simulink model "DUST4_Nonlinear_Airframe"  (R2024b)
settings: Solver=VariableStepAuto  StartTime=0.0  StopTime=10.0  RelTol=1e-3
undefined symbols (not defined in the file or in its folder): AC, Aero, mot, prop, rad, s, Vbi
libraries: aerolibasang x3, aerolibconvert2 x3, aerolibactuator x3, shared6dof x2, aerolibtransform2 x2, aerolibadyn x1, vrlib x1
(part 1 of 2)
settings Model: DataDictionary=DUST4_Airframe.sldd  Creator=Tristan  LastModifiedBy=theon

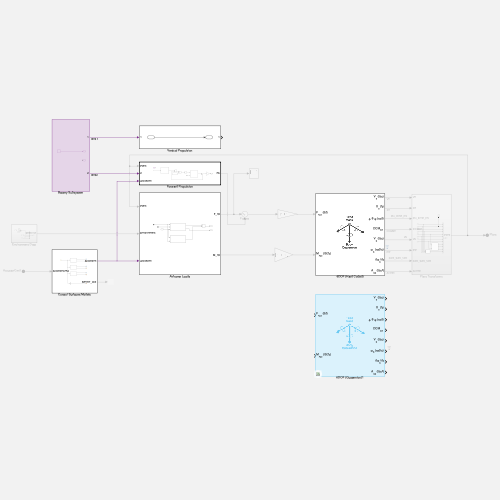
[thumbnail: Simulink's stored preview of the top-level diagram]
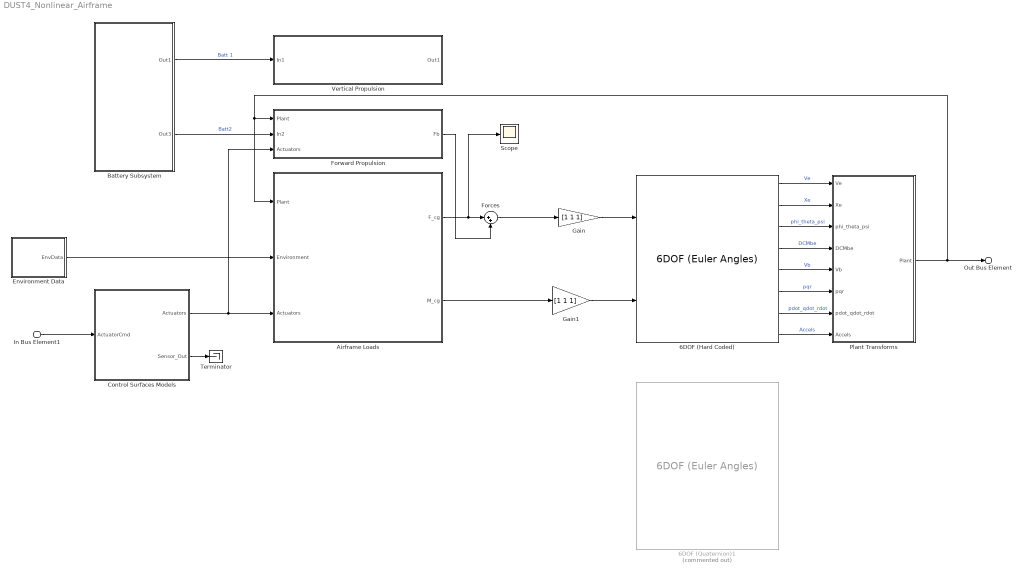
== system DUST4_Nonlinear_Airframe ==
  In Bus Element1 : Inport  PortName=ActuatorCmd
  6DOF (Hard Coded) : shared6dof/6DOF (Euler Angles)  units=English (Velocity in ft/s)  mtype=Fixed  rep=Quaternion  xme_0=[0 0 0]  Vm_0=[0 0 0]  eul_0=[0 0 0]  pm_0=[0 0 0]  mass_0=0.115  mass_e=0.5  mass_f=2.0  inertia=diag([11.38 9.6 20.40])  inertia_e=eye(3)  inertia_f=2*eye(3)  k_quat=1.0  vre_flag=on  abi_flag=off  aMode=0  xme_statename=''  Vm_statename=''  eul_statename=''  quat_statename=''  pm_statename=''  mass_statename=''
  6DOF (Quaternion)1 : shared6dof/6DOF (Euler Angles)  Commented=on  units=English (Velocity in ft/s)  mtype=Fixed  rep=Quaternion  xme_0=[0 0 0]  Vm_0=Vbi  eul_0=[0 0 0]  pm_0=[0 0 0]  mass_0=AC.mass  mass_e=0.5  mass_f=2.0  inertia=AC.Inertia  inertia_e=eye(3)  inertia_f=2*eye(3)  k_quat=1.0  vre_flag=on  abi_flag=off  aMode=0  xme_statename=''  Vm_statename=''  eul_statename=''  quat_statename=''  pm_statename=''  mass_statename=''
  Airframe Loads : Subsystem
  Battery Subsystem : Subsystem
  Control Surfaces Models : Subsystem
  Environment Data : Subsystem
  Forces : Sum  Inputs=|++
  Forward Propulsion : Subsystem  TreatAsAtomicUnit=on
  Gain : Gain  Gain=[1 1 1]
  Gain1 : Gain  Gain=[1 1 1]
  Plant Transforms : Subsystem
  Scope : Scope
  Terminator : Terminator
  Vertical Propulsion : Subsystem
  Out Bus Element : Outport  PortName=Plant
  wires:
  Forces/1 -> Gain/1
  6DOF (Hard Coded)/7 -> Plant Transforms/7(pdot_qdot_rdot)  "pdot_qdot_rdot"
  6DOF (Hard Coded)/2 -> Plant Transforms/2(Xe)  "Xe"
  6DOF (Hard Coded)/6 -> Plant Transforms/6(pqr)  "pqr"
  Airframe Loads/1(F_cg) -> Scope/1, Forces/1
  6DOF (Hard Coded)/5 -> Plant Transforms/5(Vb)  "Vb"
  In Bus Element1/1 -> Control Surfaces Models/1(ActuatorCmd)
  Environment Data/1(EnvData) -> Airframe Loads/2(Environment)
  Plant Transforms/1(Plant) -> Out Bus Element/1, Airframe Loads/1(Plant), Forward Propulsion/1(Plant)
  6DOF (Hard Coded)/3 -> Plant Transforms/3(phi_theta_psi)  "phi_theta_psi"
  6DOF (Hard Coded)/8 -> Plant Transforms/8(Accels)  "Accels"
  6DOF (Hard Coded)/1 -> Plant Transforms/1(Ve)  "Ve"
  Airframe Loads/2(M_cg) -> Gain1/1
  Gain/1 -> 6DOF (Hard Coded)/1
  Forward Propulsion/1(Fb) -> Forces/2
  6DOF (Hard Coded)/4 -> Plant Transforms/4(DCMbe)  "DCMbe"
  Control Surfaces Models/2(Sensor_Out) -> Terminator/1
  Gain1/1 -> 6DOF (Hard Coded)/2
  Battery Subsystem/2(Out3) -> Forward Propulsion/2(In2)  "Batt2"
  Battery Subsystem/1(Out1) -> Vertical Propulsion/1(In1)  "Batt 1"
  Control Surfaces Models/1(Actuators) -> Airframe Loads/3(Actuators), Forward Propulsion/3(Actuators)

== system DUST4_Nonlinear_Airframe/Airframe Loads ==
  Plant : Inport
  In Bus Element : Inport  Port=2  PortName=Environment
  In Bus Element1 : Inport  Port=3  PortName=Actuators
  Add : Sum
  Aerodynamic Loads : Subsystem
  Gravity Force : Subsystem
  F_cg : Outport
  M_cg : Outport  Port=2
  wires:
  Plant/1 -> Gravity Force/1(Plant), Aerodynamic Loads/3(plant)
  In Bus Element/1 -> Gravity Force/2(Environment), Aerodynamic Loads/1(EnvData)
  In Bus Element1/1 -> Aerodynamic Loads/2(Actuators)
  Aerodynamic Loads/1(Fb) -> Add/1
  Add/1 -> F_cg/1
  Aerodynamic Loads/2(Mb) -> M_cg/1
  Gravity Force/1(Fg_b) -> Add/2

== system DUST4_Nonlinear_Airframe/Battery Subsystem ==
  Initial Voltage : Constant
  Out1 : Outport
  Out3 : Outport  Port=2
  wires:
  Initial Voltage/1 -> Out1/1

== system DUST4_Nonlinear_Airframe/Control Surfaces Models ==
  In Bus Element1 : Inport  PortName=ActuatorCmd
  Ailerons : Subsystem
  Bus Selector : BusSelector  OutputSignals=Throttle
  Elevator : Subsystem
  Rudder : Subsystem
  Out Bus Element2 : Outport  VectorParamsAs1DForOutWhenUnconnected=off  PortName=Actuators  Element=Aileron
  Out Bus Element3 : Outport  VectorParamsAs1DForOutWhenUnconnected=off  PortName=Actuators  Element=Elevator
  Out Bus Element4 : Outport  VectorParamsAs1DForOutWhenUnconnected=off  PortName=Actuators  Element=Rudder
  BusElementOut : Outport  PortName=Actuators  Element=Throttle
  Out Bus Element12 : Outport  Port=2  VectorParamsAs1DForOutWhenUnconnected=off  PortName=Sensor_Out  Element=Ail
  Out Bus Element1 : Outport  Port=2  VectorParamsAs1DForOutWhenUnconnected=off  PortName=Sensor_Out  Element=Ele
  Out Bus Element5 : Outport  Port=2  VectorParamsAs1DForOutWhenUnconnected=off  PortName=Sensor_Out  Element=Rud
  wires:
  Ailerons/1(SensorOut) -> Out Bus Element12/1  "Rudder"
  Ailerons/2(Positions) -> Out Bus Element2/1  "Rudder"
  In Bus Element1/1 -> Bus Selector/1, Rudder/1(Commands), Elevator/1(Commands), Ailerons/1(Commands)
  Elevator/1(SensorOut) -> Out Bus Element1/1  "Rudder"
  Elevator/2(Positions) -> Out Bus Element3/1  "Rudder"
  Rudder/2(Positions) -> Out Bus Element4/1  "Rudder"
  Rudder/1(SensorOut) -> Out Bus Element5/1  "Rudder"
  Bus Selector/1 -> BusElementOut/1  "<Throttle>"

== system DUST4_Nonlinear_Airframe/Environment Data ==
  Air Density : Constant  Value=0.002377
  Bus Creator : BusCreator  Inputs=5
  Constant : Constant  Value=0
  Constant1 : Constant  Value=0
  Constant2 : Constant  Value=32.2
  Gravity Acceleration : Constant  Value=[0 0 32.2]
  Mux : Mux  Inputs=3
  Speed of Sound : Constant  Value=1100
  Wind Angular Rates : Constant  Value=[0 0 0]
  Wind Velocity : Constant  Value=[0 0 0]
  EnvData : Outport
  wires:
  Air Density/1 -> Bus Creator/3  "rho"
  Speed of Sound/1 -> Bus Creator/2  "a"
  Mux/1 -> Bus Creator/1  "Ag"
  Wind Velocity/1 -> Bus Creator/4  "WindVelocity"
  Wind Angular Rates/1 -> Bus Creator/5  "WindAngularRates"
  Bus Creator/1 -> EnvData/1  "Environment"
  Constant/1 -> Mux/1
  Constant1/1 -> Mux/2
  Constant2/1 -> Mux/3

== system DUST4_Nonlinear_Airframe/Forward Propulsion ==
  In Bus Element2 : Inport  PortName=Plant  Element=Airspeed
  In2 : Inport  Port=2
  In Bus Element1 : Inport  Port=3  PortName=Actuators  Element=Throttle
  Bus Selector1 : BusSelector  OutputSignals=Thrust,Torque
  Divide1 : Product  Inputs=*/
  Gain1 : Gain  Gain=[1 0 0]
  Integrator : Integrator  InitialCondition=200
  Motor Model : Subsystem
  Prop MOI (slug-ft^2) : Constant  Value=prop.MOI
  Propeller Model : Subsystem
  Subtract : Sum  Inputs=+-
  Fb : Outport
  wires:
  In Bus Element2/1 -> Propeller Model/2(Airspeed)
  Propeller Model/1(Propulsion Data) -> Bus Selector1/1
  Prop MOI (slug-ft^2)/1 -> Divide1/2
  Divide1/1 -> Integrator/1  "Omega dot"
  In Bus Element1/1 -> Motor Model/1(Throttle)
  Integrator/1 -> Propeller Model/1(Omega)  "omega"
  Subtract/1 -> Divide1/1
  Motor Model/1(Torque (ft-lbf)) -> Subtract/1
  Bus Selector1/2 -> Subtract/2  "<Torque>"
  Bus Selector1/1 -> Gain1/1  "<Thrust>"
  Gain1/1 -> Fb/1

== system DUST4_Nonlinear_Airframe/Plant Transforms ==
  Ve : Inport
  Xe : Inport  Port=2
  phi_theta_psi : Inport  Port=3
  DCMbe : Inport  Port=4
  Vb : Inport  Port=5
  pqr : Inport  Port=6
  pdot_qdot_rdot : Inport  Port=7
  Accels : Inport  Port=8
  ModelBus : BusCreator  Inputs=12
  Scope : Scope
  Subsystem1 : Subsystem
  WingConnectorPlant : Subsystem
  Plant : Outport
  wires:
  Ve/1 -> WingConnectorPlant/2(Ve), ModelBus/1  "Ve"
  ModelBus/1 -> Plant/1
  DCMbe/1 -> ModelBus/4, WingConnectorPlant/1(DCMbe)  "DCMbe"
  pqr/1 -> WingConnectorPlant/4(pqr), ModelBus/6  "pqr"
  pdot_qdot_rdot/1 -> ModelBus/7  "pdot_qdot_rdot"
  Subsystem1/2("alpha_dot, beta_dot") -> ModelBus/10  "alphadot_betadot"
  WingConnectorPlant/1(WingConnector) -> ModelBus/12  "AC1_Connector"
  Xe/1 -> WingConnectorPlant/3(Xe), ModelBus/2, Scope/1  "Xe"
  Subsystem1/1("alpha, beta") -> ModelBus/9  "alpha_beta"
  phi_theta_psi/1 -> ModelBus/3  "phi_theta_psi"
  Accels/1 -> Subsystem1/2(Ab), ModelBus/8  "Ab"
  Vb/1 -> Subsystem1/1(Vb), ModelBus/5  "Vb"
  Subsystem1/3(Airspeed) -> ModelBus/11  "Airspeed"

== system DUST4_Nonlinear_Airframe/Vertical Propulsion ==
  In1 : Inport
  Out1 : Outport
  wires:
  In1/1 -> Out1/1

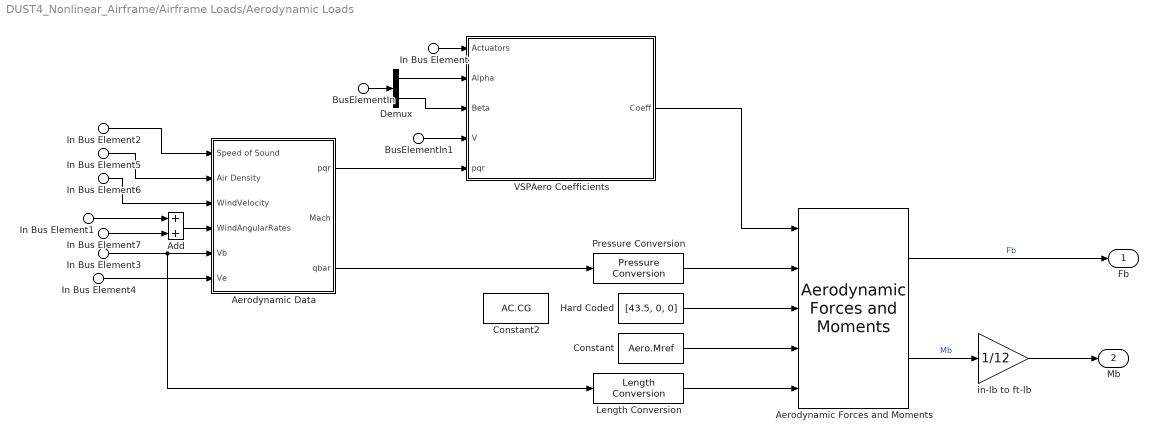
== system DUST4_Nonlinear_Airframe/Airframe Loads/Aerodynamic Loads ==
  In Bus Element6 : Inport  PortName=EnvData  Element=WindVelocity
  In Bus Element7 : Inport  PortName=EnvData  Element=WindAngularRates
  In Bus Element2 : Inport  PortName=EnvData  Element=a
  In Bus Element5 : Inport  PortName=EnvData  Element=rho
  In Bus Element : Inport  Port=2  PortName=Actuators
  In Bus Element3 : Inport  Port=3  PortName=plant  Element=Vb
  In Bus Element4 : Inport  Port=3  PortName=plant  Element=Ve
  In Bus Element1 : Inport  Port=3  PortName=plant  Element=pqr
  BusElementIn : Inport  Port=3  PortName=plant  Element=alpha_beta
  BusElementIn1 : Inport  Port=3  PortName=plant  Element=Airspeed
  Add : Sum
  Aerodynamic Forces and Moments : aerolibadyn/Aerodynamic Forces and Moments   inputAxes=Wind  outputForceAxes=Body  outputMomentAxes=Body  S=Aero.Sref  b=Aero.bref  cbar=Aero.Cref
  Aerodynamic Data : Subsystem
  Constant : Constant  Value=Aero.Mref
  Constant2 : Constant  Value=AC.CG
  Demux : Demux  Outputs=2
  Hard Coded : Constant  Value=[43.5, 0, 0]
  Length Conversion : aerolibconvert2/Length Conversion  IU=ft  OU=in
  Pressure Conversion : aerolibconvert2/Pressure Conversion  IU=psf  OU=psi
  VSPAero Coefficients : Subsystem
  in-lb to ft-lb : Gain  Gain=1/12
  Fb : Outport  VectorParamsAs1DForOutWhenUnconnected=off
  Mb : Outport  Port=2  VectorParamsAs1DForOutWhenUnconnected=off
  wires:
  In Bus Element6/1 -> Aerodynamic Data/3(WindVelocity)
  Aerodynamic Data/1("pqr ") -> VSPAero Coefficients/5(pqr)
  Aerodynamic Forces and Moments/2 -> in-lb to ft-lb/1  "Mb"
  VSPAero Coefficients/1(Coeff) -> Aerodynamic Forces and Moments/1
  In Bus Element7/1 -> Add/2
  Constant/1 -> Aerodynamic Forces and Moments/4
  In Bus Element5/1 -> Aerodynamic Data/2(Air Density)
  In Bus Element2/1 -> Aerodynamic Data/1(Speed of Sound)
  Add/1 -> Aerodynamic Data/4(WindAngularRates)
  In Bus Element4/1 -> Aerodynamic Data/6(Ve)
  Aerodynamic Forces and Moments/1 -> Fb/1  "Fb"
  In Bus Element1/1 -> Add/1
  In Bus Element/1 -> VSPAero Coefficients/1(Actuators)
  BusElementIn1/1 -> VSPAero Coefficients/4(V)
  BusElementIn/1 -> Demux/1
  Demux/1 -> VSPAero Coefficients/2(Alpha)
  Demux/2 -> VSPAero Coefficients/3(Beta)
  In Bus Element3/1 -> Length Conversion/1, Aerodynamic Data/5(Vb)
  Aerodynamic Data/3(qbar) -> Pressure Conversion/1
  Hard Coded/1 -> Aerodynamic Forces and Moments/3
  Pressure Conversion/1 -> Aerodynamic Forces and Moments/2
  Length Conversion/1 -> Aerodynamic Forces and Moments/5
  in-lb to ft-lb/1 -> Mb/1

== system DUST4_Nonlinear_Airframe/Airframe Loads/Gravity Force ==
  Plant : Inport
  Bus Element In2 : Inport  Port=2  PortName=Environment
  Acc to Force : Gain  Gain=AC.mass  OutDataTypeStr=Inherit: Same as input  ParamDataTypeStr=Inherit: Same as input
  Bus Selector : BusSelector  OutputSignals=DCMbe
  Bus Selector1 : BusSelector  OutputSignals=Ag
  Constant : Constant  Value=[0 0 32.2]
  Fg_body : Product  Multiplication=Matrix(*)
  Fg_b : Outport
  wires:
  Bus Selector/1 -> Fg_body/1  "<DCMbe>"
  Acc to Force/1 -> Fg_body/2
  Plant/1 -> Bus Selector/1
  Bus Element In2/1 -> Bus Selector1/1
  Bus Selector1/1 -> ?  "<Ag>"
  Fg_body/1 -> Fg_b/1
  Constant/1 -> Acc to Force/1

== system DUST4_Nonlinear_Airframe/Control Surfaces Models/Ailerons ==
  In Bus Element4 : Inport  PortName=Commands  Element=Aileron
  Nonlinear Second-Order Actuator1 : aerolibactuator/Nonlinear Second-Order Actuator  wn_fin=10  z_fin=1  fin_max=20*pi/180  fin_min=-20*pi/180  fin_maxrate=90*pi/180  fin_act_0=0  fin_act_vel=0
  Scope : Scope  NumInputPorts=2
  SensorOut : Outport  VectorParamsAs1DForOutWhenUnconnected=off
  Positions : Outport  Port=2  VectorParamsAs1DForOutWhenUnconnected=off
  wires:
  Nonlinear Second-Order Actuator1/1 -> Positions/1, Scope/2, SensorOut/1
  In Bus Element4/1 -> Scope/1, Nonlinear Second-Order Actuator1/1  "Ail"

== system DUST4_Nonlinear_Airframe/Control Surfaces Models/Elevator ==
  In Bus Element4 : Inport  PortName=Commands  Element=Elevator
  Nonlinear Second-Order Actuator1 : aerolibactuator/Nonlinear Second-Order Actuator  wn_fin=10  z_fin=1  fin_max=20*pi/180  fin_min=-20*pi/180  fin_maxrate=90*pi/180  fin_act_0=0  fin_act_vel=0
  SensorOut : Outport  VectorParamsAs1DForOutWhenUnconnected=off
  Positions : Outport  Port=2  VectorParamsAs1DForOutWhenUnconnected=off
  wires:
  Nonlinear Second-Order Actuator1/1 -> Positions/1, SensorOut/1
  In Bus Element4/1 -> Nonlinear Second-Order Actuator1/1  "Ele"

== system DUST4_Nonlinear_Airframe/Control Surfaces Models/Rudder ==
  In Bus Element4 : Inport  PortName=Commands  Element=Rudder
  Nonlinear Second-Order Actuator1 : aerolibactuator/Nonlinear Second-Order Actuator  wn_fin=10  z_fin=1  fin_max=20*pi/180  fin_min=-20*pi/180  fin_maxrate=90*pi/180  fin_act_0=0  fin_act_vel=0
  SensorOut : Outport  VectorParamsAs1DForOutWhenUnconnected=off
  Positions : Outport  Port=2  VectorParamsAs1DForOutWhenUnconnected=off
  wires:
  Nonlinear Second-Order Actuator1/1 -> Positions/1, SensorOut/1
  In Bus Element4/1 -> Nonlinear Second-Order Actuator1/1  "Rud"

== system DUST4_Nonlinear_Airframe/Forward Propulsion/Motor Model ==
  Throttle : Inport
  Divide : Product  Inputs=*/
  Kv (RPM/V) : Constant  Value=mot.Kv
  Max Current : Gain  Gain=mot.amp
  Mot Efficiency : Gain
  Motor Conversion Constant : Gain  Gain=8.3
  SI Conversion : Gain  Gain=.7376
  Torque (ft-lbf) : Outport
  wires:
  Mot Efficiency/1 -> Torque (ft-lbf)/1  "Torque (ft-lbf)"
  Throttle/1 -> Max Current/1
  Kv (RPM/V)/1 -> Divide/2
  Divide/1 -> Motor Conversion Constant/1
  Max Current/1 -> Divide/1
  Motor Conversion Constant/1 -> SI Conversion/1  "Torque (N.m)"
  SI Conversion/1 -> Mot Efficiency/1  "Torque (ft-lbf)"

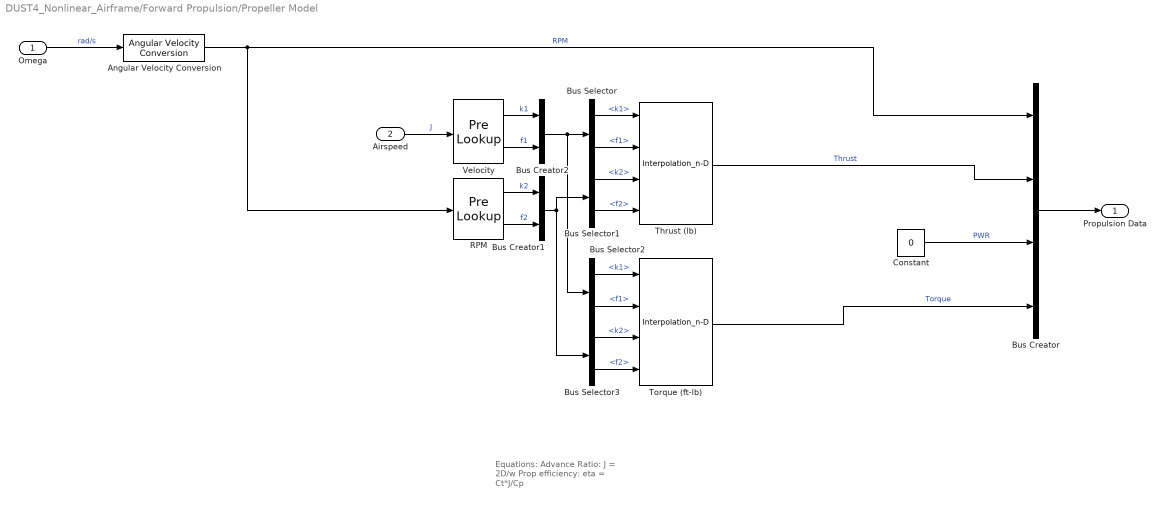
== system DUST4_Nonlinear_Airframe/Forward Propulsion/Propeller Model ==
  note: Equations:
      |
      | Advance Ratio: J = 2D/w
      | Prop efficiency: eta = Ct*J/Cp
  Omega : Inport
  Airspeed : Inport  Port=2
  Angular Velocity Conversion : aerolibconvert2/Angular Velocity Conversion  IU=rad/s  OU=rpm
  Bus Creator : BusCreator  Inputs=4
  Bus Creator1 : BusCreator  Inputs=2
  Bus Creator2 : BusCreator  Inputs=2
  Bus Selector : BusSelector  OutputSignals=k1,f1
  Bus Selector1 : BusSelector  OutputSignals=k2,f2
  Bus Selector2 : BusSelector  OutputSignals=k1,f1
  Bus Selector3 : BusSelector  OutputSignals=k2,f2
  Constant : Constant  Value=0
  RPM : PreLookup  BreakpointsData=prop.RPM  ExtrapMethod=Linear
  Thrust (lb) : Interpolation_n-D  Table=prop.Thrust  InternalRulePriority=Speed
  Torque (ft-lb) : Interpolation_n-D  Table=prop.Torque  ExtrapMethod=Clip  InternalRulePriority=Speed
  Velocity : PreLookup  BreakpointsData=prop.vel
  Propulsion Data : Outport
  wires:
  Constant/1 -> Bus Creator/3  "PWR"
  Torque (ft-lb)/1 -> Bus Creator/4  "Torque"
  Angular Velocity Conversion/1 -> RPM/1, Bus Creator/1  "RPM"
  Bus Creator/1 -> Propulsion Data/1
  Omega/1 -> Angular Velocity Conversion/1  "rad/s"
  Airspeed/1 -> Velocity/1  "J"
  Velocity/2 -> Bus Creator2/2  "f1"
  Bus Creator2/1 -> Bus Selector/1, Bus Selector2/1
  Bus Creator1/1 -> Bus Selector1/1, Bus Selector3/1
  Velocity/1 -> Bus Creator2/1  "k1"
  Bus Selector2/2 -> Torque (ft-lb)/2  "<f1>"
  RPM/1 -> Bus Creator1/1  "k2"
  Bus Selector2/1 -> Torque (ft-lb)/1  "<k1>"
  RPM/2 -> Bus Creator1/2  "f2"
  Thrust (lb)/1 -> Bus Creator/2  "Thrust"
  Bus Selector/2 -> Thrust (lb)/2  "<f1>"
  Bus Selector3/2 -> Torque (ft-lb)/4  "<f2>"
  Bus Selector/1 -> Thrust (lb)/1  "<k1>"
  Bus Selector1/2 -> Thrust (lb)/4  "<f2>"
  Bus Selector3/1 -> Torque (ft-lb)/3  "<k2>"
  Bus Selector1/1 -> Thrust (lb)/3  "<k2>"

== system DUST4_Nonlinear_Airframe/Plant Transforms/Subsystem1 ==
  Vb : Inport
  Ab : Inport  Port=2
  Direction Cosine Matrix Body to Wind : aerolibtransform2/Direction Cosine Matrix Body to Wind
  "Incidence, Sideslip, & Airspeed" : aerolibasang/Incidence, Sideslip, & Airspeed
  Memory4 : Memory  InitialCondition=Vbi
  Mux4 : Mux  Inputs=2
  Product1 : Product  Multiplication=Matrix(*)  InputSameDT=on  SaturateOnIntegerOverflow=on  OutDataTypeStr=Inherit: Same as first input
  "calc alpha_dot, beta_dot" : Subsystem
  "alpha, beta" : Outport  Unit=rad  VectorParamsAs1DForOutWhenUnconnected=off
  "alpha_dot, beta_dot" : Outport  Port=2  Unit=rad/s  VectorParamsAs1DForOutWhenUnconnected=off
  Airspeed : Outport  Port=3
  wires:
  "Incidence, Sideslip, & Airspeed"/2 -> Mux4/2
  Mux4/1 -> "alpha, beta"/1, Direction Cosine Matrix Body to Wind/1, "calc alpha_dot, beta_dot"/1(alpha,beta)
  Direction Cosine Matrix Body to Wind/1 -> Product1/1
  "Incidence, Sideslip, & Airspeed"/1 -> Mux4/1
  Memory4/1 -> Product1/2, "Incidence, Sideslip, & Airspeed"/1
  Product1/1 -> "calc alpha_dot, beta_dot"/3(Vw)
  Ab/1 -> "calc alpha_dot, beta_dot"/2(Ab)
  "Incidence, Sideslip, & Airspeed"/3 -> Airspeed/1
  "calc alpha_dot, beta_dot"/1("alpha_dot, beta_dot") -> "alpha_dot, beta_dot"/1
  Vb/1 -> Memory4/1

== system DUST4_Nonlinear_Airframe/Plant Transforms/WingConnectorPlant ==
  note: Give Position of Line Connection Point
  DCMbe : Inport
  Ve : Inport  Port=2
  Xe : Inport  Port=3
  pqr : Inport  Port=4
  Add1 : Sum
  Add2 : Sum
  Body2Earth : Product  Multiplication=Matrix(*)
  Bus Creator : BusCreator  Inputs=2
  Cross Product : vrlib/Utilities/Cross Product
  Matrix Multiply1 : Product  Multiplication=Matrix(*)
  Tether DCG : Constant  Value=[0 0 0]
  Transpose : Math  Operator=transpose
  WingConnector : Outport
  wires:
  Bus Creator/1 -> WingConnector/1
  Transpose/1 -> Body2Earth/1, Matrix Multiply1/1
  Body2Earth/1 -> Add1/1
  Add2/1 -> Bus Creator/2  "Ve"
  Xe/1 -> Add1/2
  Matrix Multiply1/1 -> Add2/1
  Tether DCG/1 -> Cross Product/2, Body2Earth/2
  pqr/1 -> Cross Product/1
  Cross Product/1 -> Matrix Multiply1/2
  Add1/1 -> Bus Creator/1  "Xe"
  DCMbe/1 -> Transpose/1
  Ve/1 -> Add2/2

== system DUST4_Nonlinear_Airframe/Airframe Loads/Aerodynamic Loads/Aerodynamic Data ==
  note: TODO: clean up interface
  Speed of Sound : Inport
  Air Density : Inport  Port=2
  WindVelocity : Inport  Port=3  PortDimensions=3
  WindAngularRates : Inport  Port=4  PortDimensions=3
  Vb : Inport  Port=5  PortDimensions=3
  Ve : Inport  Port=6  PortDimensions=3
  Dynamic Pressure : aerolibasang/Dynamic Pressure
  Mach Number : aerolibasang/Mach Number
  Sum2 : Sum  Inputs=|+-  InputSameDT=on  SaturateOnIntegerOverflow=on  OutDataTypeStr=Inherit: Same as first input
  Terminator : Terminator
  "pqr " : Outport  VectorParamsAs1DForOutWhenUnconnected=off
  Mach : Outport  Port=2  VectorParamsAs1DForOutWhenUnconnected=off
  qbar : Outport  Port=3  VectorParamsAs1DForOutWhenUnconnected=off
  wires:
  Dynamic Pressure/1 -> qbar/1  "qbar"
  Sum2/1 -> Mach Number/1, Dynamic Pressure/1
  Ve/1 -> Terminator/1
  Mach Number/1 -> Mach/1  "Mach"
  WindVelocity/1 -> Sum2/2
  Air Density/1 -> Dynamic Pressure/2
  WindAngularRates/1 -> "pqr "/1
  Speed of Sound/1 -> Mach Number/2
  Vb/1 -> Sum2/1

== system DUST4_Nonlinear_Airframe/Airframe Loads/Aerodynamic Loads/VSPAero Coefficients ==
  Actuators : Inport
  Alpha : Inport  Port=2  Unit=rad
  Beta : Inport  Port=3  Unit=rad
  V : Inport  Port=4
  pqr : Inport  Port=5
  Actuator Effects : Subsystem
  Fuselage Effects : Subsystem  Commented=on
  Sum : Sum  Inputs=|+++
  Wing Effects : Subsystem
  Wing Rate Effects : Subsystem
  alpha_rad : UnitConversion
  beta_rad : UnitConversion
  Coeff : Outport  VectorParamsAs1DForOutWhenUnconnected=off
  wires:
  Wing Rate Effects/1(cl) -> Sum/3
  Sum/1 -> Coeff/1
  Wing Effects/1(coeffs) -> Sum/1
  alpha_rad/1 -> Wing Rate Effects/1(Alpha), Actuator Effects/1(Alpha), Wing Effects/1(Alpha)
  Actuators/1 -> Actuator Effects/3("Actuator Deflections ")
  V/1 -> Wing Rate Effects/4(V)
  Alpha/1 -> alpha_rad/1
  beta_rad/1 -> Actuator Effects/2(Beta), Wing Rate Effects/2(Beta), Wing Effects/2(Beta)
  Beta/1 -> beta_rad/1
  Actuator Effects/1(coeffs) -> Sum/2
  pqr/1 -> Wing Rate Effects/3(pqr)

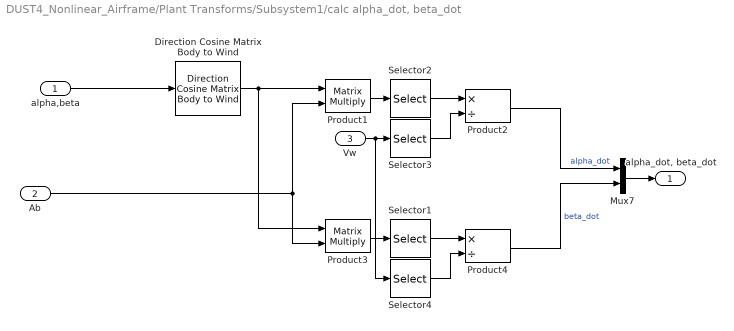
== system DUST4_Nonlinear_Airframe/Plant Transforms/Subsystem1/calc alpha_dot, beta_dot ==
  alpha,beta : Inport
  Ab : Inport  Port=2
  Vw : Inport  Port=3
  Direction Cosine Matrix Body to Wind : aerolibtransform2/Direction Cosine Matrix Body to Wind
  Mux7 : Mux  Inputs=2
  Product1 : Product  Multiplication=Matrix(*)  InputSameDT=on  SaturateOnIntegerOverflow=on  OutDataTypeStr=Inherit: Same as first input
  Product2 : Product  Inputs=*/  InputSameDT=on  SaturateOnIntegerOverflow=on  OutDataTypeStr=Inherit: Same as first input
  Product3 : Product  Multiplication=Matrix(*)  InputSameDT=on  SaturateOnIntegerOverflow=on  OutDataTypeStr=Inherit: Same as first input
  Product4 : Product  Inputs=*/  InputSameDT=on  SaturateOnIntegerOverflow=on  OutDataTypeStr=Inherit: Same as first input
  Selector1 : Selector  IndexMode=Zero-based  InputPortWidth=3  IndexOptions=Index vector (dialog)  Indices=1  OutputSizes=1
  Selector2 : Selector  IndexMode=Zero-based  InputPortWidth=3  IndexOptions=Index vector (dialog)  Indices=2  OutputSizes=1
  Selector3 : Selector  IndexMode=Zero-based  InputPortWidth=3  IndexOptions=Index vector (dialog)  Indices=0  OutputSizes=1
  Selector4 : Selector  IndexMode=Zero-based  InputPortWidth=3  IndexOptions=Index vector (dialog)  Indices=0  OutputSizes=1
  "alpha_dot, beta_dot" : Outport  VectorParamsAs1DForOutWhenUnconnected=off
  wires:
  Product1/1 -> Selector2/1
  Selector2/1 -> Product2/1
  Selector3/1 -> Product2/2
  alpha,beta/1 -> Direction Cosine Matrix Body to Wind/1
  Product2/1 -> Mux7/1  "alpha_dot"
  Ab/1 -> Product1/2, Product3/2
  Vw/1 -> Selector4/1, Selector3/1
  Product4/1 -> Mux7/2  "beta_dot"
  Direction Cosine Matrix Body to Wind/1 -> Product3/1, Product1/1
  Selector1/1 -> Product4/1
  Selector4/1 -> Product4/2
  Product3/1 -> Selector1/1
  Mux7/1 -> "alpha_dot, beta_dot"/1

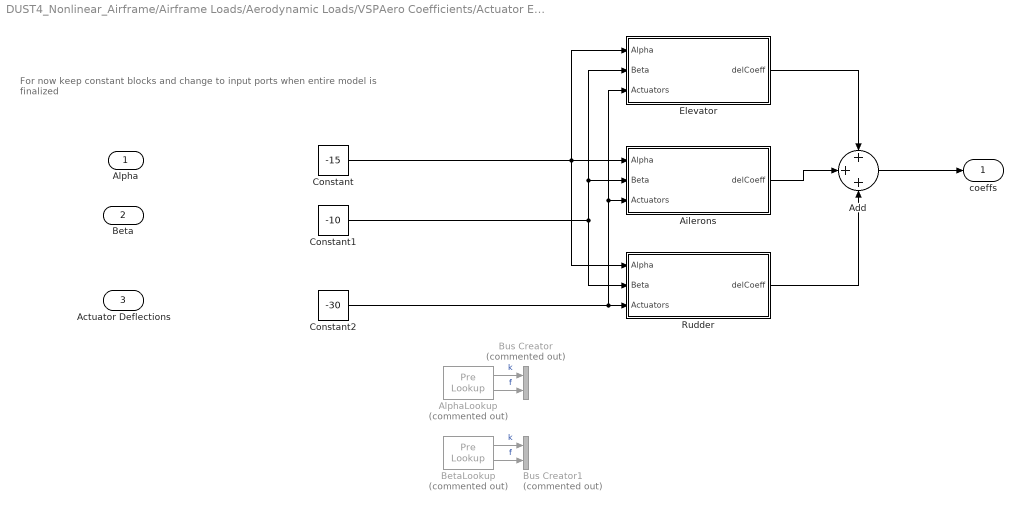
== system DUST4_Nonlinear_Airframe/Airframe Loads/Aerodynamic Loads/VSPAero Coefficients/Actuator Effects ==
  note: For now keep
      | constant blocks and change to input ports when entire model is finalized
  Alpha : Inport  Unit=deg
  Beta : Inport  Port=2  Unit=deg
  "Actuator Deflections " : Inport  Port=3
  Add : Sum  Inputs=+++
  Ailerons : Subsystem
  AlphaLookup : PreLookup  Commented=on  BreakpointsData=Aero.alpha_vec  BeginIndexSearchUsingPreviousIndexResult=on  ExtrapMethod=Linear
  BetaLookup : PreLookup  Commented=on  BreakpointsData=Aero.beta_vec  BeginIndexSearchUsingPreviousIndexResult=on  ExtrapMethod=Linear
  Bus Creator : BusCreator  Commented=on  Inputs=2
  Bus Creator1 : BusCreator  Commented=on  Inputs=2
  Constant : Constant  Value=-15
  Constant1 : Constant  Value=-10
  Constant2 : Constant  Value=-30
  Elevator : Subsystem
  Rudder : Subsystem
  coeffs : Outport  VectorParamsAs1DForOutWhenUnconnected=off
  wires:
  Add/1 -> coeffs/1
  Ailerons/1(delCoeff) -> Add/2
  Constant1/1 -> Rudder/2(Beta), Ailerons/2(Beta), Elevator/2(Beta)
  BetaLookup/2 -> Bus Creator1/2  "f"
  AlphaLookup/2 -> Bus Creator/2  "f"
  AlphaLookup/1 -> Bus Creator/1  "k"
  Constant2/1 -> Ailerons/3(Actuators), Elevator/3(Actuators), Rudder/3(Actuators)
  BetaLookup/1 -> Bus Creator1/1  "k"
  Elevator/1(delCoeff) -> Add/1
  Constant/1 -> Ailerons/1(Alpha), Elevator/1(Alpha), Rudder/1(Alpha)
  Rudder/1(delCoeff) -> Add/3

== system DUST4_Nonlinear_Airframe/Airframe Loads/Aerodynamic Loads/VSPAero Coefficients/Fuselage Effects ==
  In1 : Inport
  Out1 : Outport
  wires:
  In1/1 -> Out1/1

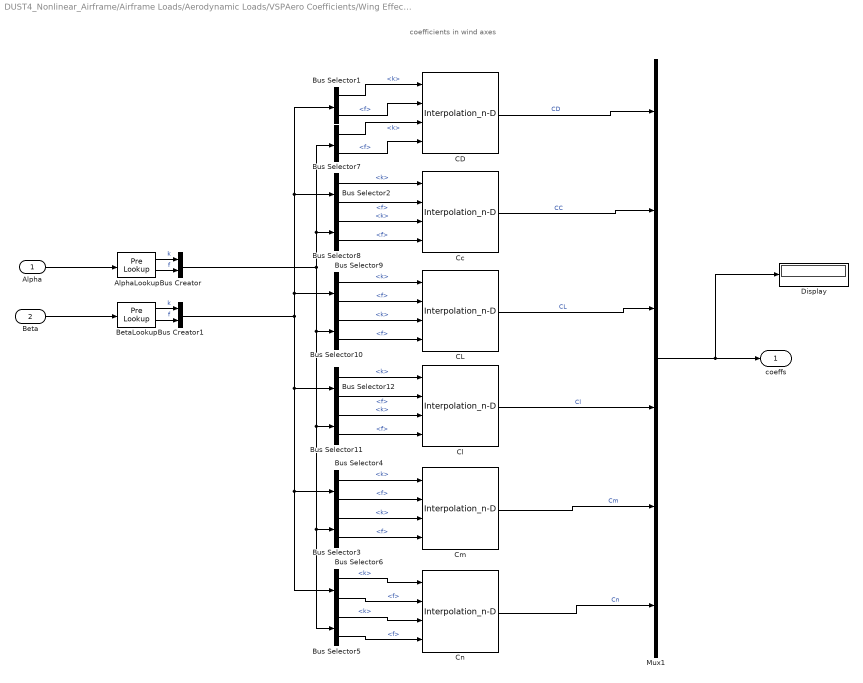
== system DUST4_Nonlinear_Airframe/Airframe Loads/Aerodynamic Loads/VSPAero Coefficients/Wing Effects ==
  note: coefficients in wind axes
  Alpha : Inport  Unit=deg
  Beta : Inport  Port=2  Unit=deg
  AlphaLookup : PreLookup  BreakpointsData=Aero.alpha_vec  BeginIndexSearchUsingPreviousIndexResult=on  ExtrapMethod=Linear
  BetaLookup : PreLookup  BreakpointsData=Aero.beta_vec  BeginIndexSearchUsingPreviousIndexResult=on  ExtrapMethod=Linear
  Bus Creator : BusCreator  Inputs=2
  Bus Creator1 : BusCreator  Inputs=2
  Bus Selector{1..12} (12 alike) : BusSelector  OutputSignals=k,f
  CD : Interpolation_n-D  Table=Aero.CD  RemoveProtectionIndex=on  SaturateOnIntegerOverflow=on
  CL : Interpolation_n-D  Table=Aero.CL  RemoveProtectionIndex=on  SaturateOnIntegerOverflow=on
  Cc : Interpolation_n-D  Table=Aero.Cc  RemoveProtectionIndex=on  SaturateOnIntegerOverflow=on
  Cl : Interpolation_n-D  Table=Aero.Cl  RemoveProtectionIndex=on  SaturateOnIntegerOverflow=on
  Cm : Interpolation_n-D  Table=Aero.Cm  RemoveProtectionIndex=on  SaturateOnIntegerOverflow=on
  Cn : Interpolation_n-D  Table=Aero.Cn  RemoveProtectionIndex=on  SaturateOnIntegerOverflow=on
  Display : Display
  Mux1 : Mux  Inputs=6
  coeffs : Outport  VectorParamsAs1DForOutWhenUnconnected=off
  wires:
  BetaLookup/2 -> Bus Creator1/2  "f"
  AlphaLookup/2 -> Bus Creator/2  "f"
  AlphaLookup/1 -> Bus Creator/1  "k"
  BetaLookup/1 -> Bus Creator1/1  "k"
  Mux1/1 -> Display/1, coeffs/1
  Beta/1 -> BetaLookup/1
  Alpha/1 -> AlphaLookup/1
  Bus Selector6/1 -> Cn/1  "<k>"
  Cm/1 -> Mux1/5  "Cm"
  Bus Selector11/1 -> Cl/3  "<k>"
  Bus Creator1/1 -> Bus Selector4/1, Bus Selector6/1, Bus Selector12/1, Bus Selector2/1, Bus Selector1/1, Bus Selector9/1
  Bus Selector8/1 -> Cc/3  "<k>"
  Bus Selector5/1 -> Cn/3  "<k>"
  Bus Selector11/2 -> Cl/4  "<f>"
  Bus Selector5/2 -> Cn/4  "<f>"
  Bus Selector7/1 -> CD/3  "<k>"
  Bus Selector4/2 -> Cm/2  "<f>"
  Bus Selector3/2 -> Cm/4  "<f>"
  Bus Selector12/1 -> Cl/1  "<k>"
  Bus Selector1/1 -> CD/1  "<k>"
  Bus Selector8/2 -> Cc/4  "<f>"
  CL/1 -> Mux1/3  "CL"
  Bus Selector12/2 -> Cl/2  "<f>"
  Bus Selector10/1 -> CL/3  "<k>"
  Bus Selector9/1 -> CL/1  "<k>"
  Bus Selector2/1 -> Cc/1  "<k>"
  Bus Selector2/2 -> Cc/2  "<f>"
  Bus Selector1/2 -> CD/2  "<f>"
  Bus Selector7/2 -> CD/4  "<f>"
  Bus Selector10/2 -> CL/4  "<f>"
  Bus Selector6/2 -> Cn/2  "<f>"
  Cn/1 -> Mux1/6  "Cn"
  Bus Selector4/1 -> Cm/1  "<k>"
  Bus Creator/1 -> Bus Selector8/1, Bus Selector7/1, Bus Selector3/1, Bus Selector5/1, Bus Selector11/1, Bus Selector10/1
  Cc/1 -> Mux1/2  "CC"
  Bus Selector9/2 -> CL/2  "<f>"
  Bus Selector3/1 -> Cm/3  "<k>"
  Cl/1 -> Mux1/4  "Cl"
  CD/1 -> Mux1/1  "CD"

== system DUST4_Nonlinear_Airframe/Airframe Loads/Aerodynamic Loads/VSPAero Coefficients/Wing Rate Effects ==
  note: Remove these look-up tables when submodels are finalized
  Alpha : Inport  Unit=deg
  Beta : Inport  Port=2  Unit=deg
  pqr : Inport  Port=3
  V : Inport  Port=4
  Aero Surfaces : Subsystem
  AlphaLookup : PreLookup  BreakpointsData=Aero.alpha_vec  BeginIndexSearchUsingPreviousIndexResult=on  ExtrapMethod=Linear
  BetaLookup : PreLookup  BreakpointsData=Aero.beta_vec  BeginIndexSearchUsingPreviousIndexResult=on  ExtrapMethod=Linear
  Bus Creator : BusCreator  Inputs=2
  Bus Creator1 : BusCreator  Inputs=2
  Scope : Scope
  cl : Outport  VectorParamsAs1DForOutWhenUnconnected=off
  wires:
  V/1 -> Aero Surfaces/4(V)
  pqr/1 -> Aero Surfaces/3(pqr)
  Bus Creator1/1 -> Aero Surfaces/2(Beta)
  BetaLookup/2 -> Bus Creator1/2  "f"
  AlphaLookup/2 -> Bus Creator/2  "f"
  AlphaLookup/1 -> Bus Creator/1  "k"
  BetaLookup/1 -> Bus Creator1/1  "k"
  Aero Surfaces/1(delCoeff) -> cl/1, Scope/1
  Beta/1 -> BetaLookup/1
  Alpha/1 -> AlphaLookup/1
  Bus Creator/1 -> Aero Surfaces/1(Alpha)

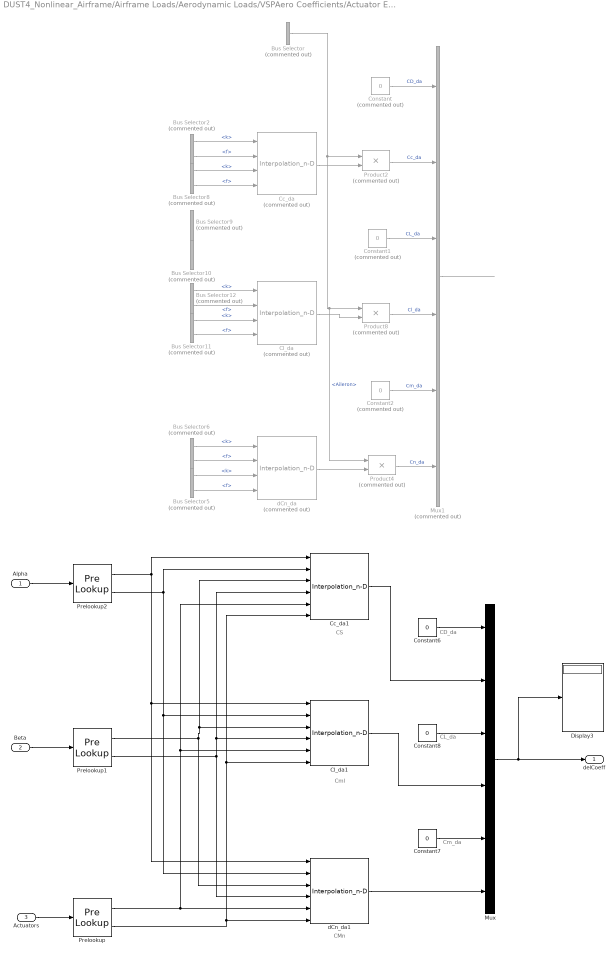
== system DUST4_Nonlinear_Airframe/Airframe Loads/Aerodynamic Loads/VSPAero Coefficients/Actuator Effects/Ailerons ==
  note: CL_da
  note: CD_da
  note: Cm_da
  note: CMn
  note: CS
  note: Cml
  Alpha : Inport
  Beta : Inport  Port=2
  Actuators : Inport  Port=3
  Bus Selector : BusSelector  Commented=on  OutputSignals=Aileron
  Bus Selector{2,5..6,8..12} (8 alike) : BusSelector  Commented=on  OutputSignals=k,f
  Cc_da : Interpolation_n-D  Commented=on  Table=Aero.Cc_da  RemoveProtectionIndex=on  SaturateOnIntegerOverflow=on
  Cc_da1 : Interpolation_n-D  NumberOfTableDimensions=3  Table=Aero.Cc_da  RemoveProtectionIndex=on  SaturateOnIntegerOverflow=on
      settings: InputPortMap=u0,u1,u2,u3,u4,u5
  Cl_da : Interpolation_n-D  Commented=on  Table=Aero.Cl_da  RemoveProtectionIndex=on  SaturateOnIntegerOverflow=on
  Cl_da1 : Interpolation_n-D  NumberOfTableDimensions=3  Table=Aero.Cl_da  RemoveProtectionIndex=on  SaturateOnIntegerOverflow=on
      settings: InputPortMap=u0,u1,u2,u3,u4,u5
  Constant : Constant  Commented=on  Value=0
  Constant1 : Constant  Commented=on  Value=0
  Constant2 : Constant  Commented=on  Value=0
  Constant6 : Constant  Value=0
  Constant7 : Constant  Value=0
  Constant8 : Constant  Value=0
  Display3 : Display
  Mux : Mux  Inputs=6
  Mux1 : Mux  Commented=on  Inputs=6
  Prelookup : PreLookup  BreakpointsData=Aero.delta_vec  ExtrapMethod=Linear
  Prelookup1 : PreLookup  BreakpointsData=Aero.beta_vec  ExtrapMethod=Linear
  Prelookup2 : PreLookup  BreakpointsData=Aero.alpha_vec  ExtrapMethod=Linear
  Product2 : Product  Commented=on  InputSameDT=on  SaturateOnIntegerOverflow=on  OutDataTypeStr=Inherit: Same as first input
  Product4 : Product  Commented=on  InputSameDT=on  SaturateOnIntegerOverflow=on  OutDataTypeStr=Inherit: Same as first input
  Product8 : Product  Commented=on  InputSameDT=on  SaturateOnIntegerOverflow=on  OutDataTypeStr=Inherit: Same as first input
  dCn_da : Interpolation_n-D  Commented=on  Table=Aero.Cn_da  RemoveProtectionIndex=on  SaturateOnIntegerOverflow=on
  dCn_da1 : Interpolation_n-D  NumberOfTableDimensions=3  Table=Aero.Cn_da  RemoveProtectionIndex=on  SaturateOnIntegerOverflow=on
      settings: InputPortMap=u0,u1,u2,u3,u4,u5
  delCoeff : Outport  VectorParamsAs1DForOutWhenUnconnected=off
  wires:
  Cc_da/1 -> Product2/2
  Mux1/1 -> ?
  Product2/1 -> Mux1/2  "Cc_da"
  Bus Selector2/1 -> Cc_da/1  "<k>"
  ? -> Bus Selector/1
  Bus Selector2/2 -> Cc_da/2  "<f>"
  Constant/1 -> Mux1/1  "CD_da"
  Bus Selector8/1 -> Cc_da/3  "<k>"
  Bus Selector8/2 -> Cc_da/4  "<f>"
  Constant1/1 -> Mux1/3  "CL_da"
  Bus Selector11/2 -> Cl_da/4  "<f>"
  Bus Selector11/1 -> Cl_da/3  "<k>"
  Bus Selector12/2 -> Cl_da/2  "<f>"
  Bus Selector12/1 -> Cl_da/1  "<k>"
  Product8/1 -> Mux1/4  "Cl_da"
  Cl_da/1 -> Product8/2
  Bus Selector5/1 -> dCn_da/3  "<k>"
  ? -> Bus Selector5/1, Bus Selector11/1, Bus Selector10/1, Bus Selector8/1
  Bus Selector5/2 -> dCn_da/4  "<f>"
  dCn_da/1 -> Product4/2
  ? -> Bus Selector6/1, Bus Selector12/1, Bus Selector2/1, Bus Selector9/1
  Bus Selector6/2 -> dCn_da/2  "<f>"
  Bus Selector/1 -> Product4/1, Product8/1, Product2/1  "<Aileron>"
  Bus Selector6/1 -> dCn_da/1  "<k>"
  Constant2/1 -> Mux1/5  "Cm_da"
  Product4/1 -> Mux1/6  "Cn_da"
  Constant7/1 -> Mux/5
  Constant6/1 -> Mux/1
  dCn_da1/1 -> Mux/6
  Beta/1 -> Prelookup1/1
  Prelookup2/1 -> dCn_da1/1, Cl_da1/1, Cc_da1/1
  Cc_da1/1 -> Mux/2
  Mux/1 -> delCoeff/1, Display3/1
  Prelookup/1 -> Cc_da1/5, Cl_da1/5, dCn_da1/5
  Prelookup/2 -> Cc_da1/6, Cl_da1/6, dCn_da1/6
  Constant8/1 -> Mux/3
  Prelookup2/2 -> dCn_da1/2, Cl_da1/2, Cc_da1/2
  Cl_da1/1 -> Mux/4
  Prelookup1/2 -> Cc_da1/4, Cl_da1/4, dCn_da1/4
  Prelookup1/1 -> Cc_da1/3, Cl_da1/3, dCn_da1/3
  Actuators/1 -> Prelookup/1
  Alpha/1 -> Prelookup2/1

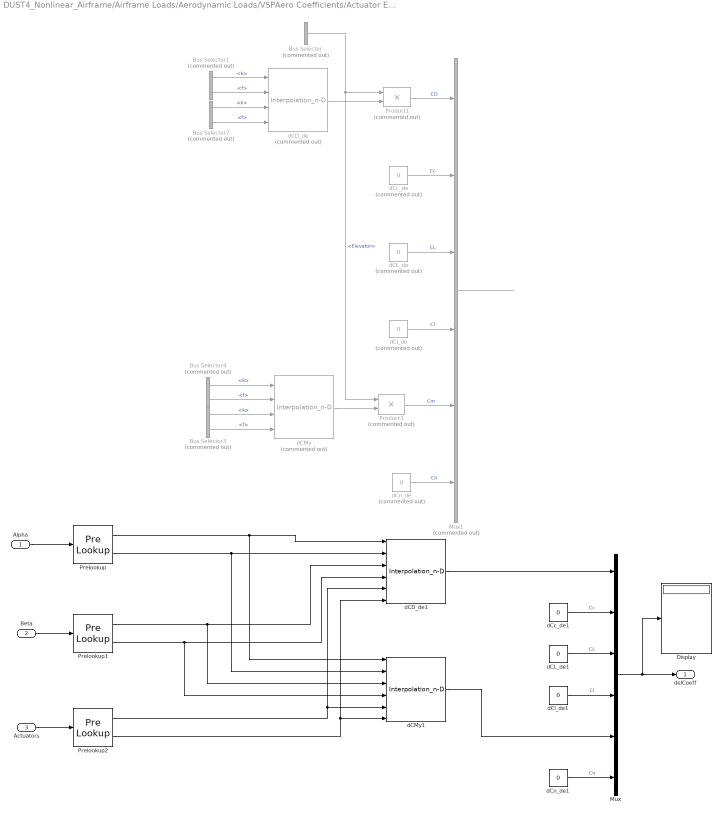
== system DUST4_Nonlinear_Airframe/Airframe Loads/Aerodynamic Loads/VSPAero Coefficients/Actuator Effects/Elevator ==
  Alpha : Inport
  Beta : Inport  Port=2
  Actuators : Inport  Port=3
  Bus Selector : BusSelector  Commented=on  OutputSignals=Elevator
  Bus Selector{1,3..4,7} (4 alike) : BusSelector  Commented=on  OutputSignals=k,f
  Display : Display
  Mux : Mux  Inputs=6
  Mux1 : Mux  Commented=on  Inputs=6
  Prelookup : PreLookup  BreakpointsData=Aero.alpha_vec  ExtrapMethod=Linear
  Prelookup1 : PreLookup  BreakpointsData=Aero.beta_vec  ExtrapMethod=Linear
  Prelookup2 : PreLookup  BreakpointsData=Aero.delta_vec  ExtrapMethod=Linear
  Product1 : Product  Commented=on  InputSameDT=on  SaturateOnIntegerOverflow=on  OutDataTypeStr=Inherit: Same as first input
  Product3 : Product  Commented=on  InputSameDT=on  SaturateOnIntegerOverflow=on  OutDataTypeStr=Inherit: Same as first input
  dCD_de : Interpolation_n-D  Commented=on  Table=Aero.CD_de  RemoveProtectionIndex=on  SaturateOnIntegerOverflow=on
  dCD_de1 : Interpolation_n-D  NumberOfTableDimensions=3  Table=Aero.CD_de  RemoveProtectionIndex=on  SaturateOnIntegerOverflow=on
      settings: InputPortMap=u0,u1,u2,u3,u4,u5
  dCL_de : Constant  Commented=on  Value=0
  dCL_de1 : Constant  Value=0
  dCMy : Interpolation_n-D  Commented=on  Table=Aero.Cm_de  RemoveProtectionIndex=on  SaturateOnIntegerOverflow=on
  dCMy1 : Interpolation_n-D  NumberOfTableDimensions=3  Table=Aero.Cm_de  RemoveProtectionIndex=on  SaturateOnIntegerOverflow=on
      settings: InputPortMap=u0,u1,u2,u3,u4,u5
  dCc_de : Constant  Commented=on  Value=0
  dCc_de1 : Constant  Value=0
  dCl_de : Constant  Commented=on  Value=0
  dCl_de1 : Constant  Value=0
  dCn_de : Constant  Commented=on  Value=0
  dCn_de1 : Constant  Value=0
  delCoeff : Outport  VectorParamsAs1DForOutWhenUnconnected=off
  wires:
  Mux1/1 -> ?
  Bus Selector1/2 -> dCD_de/2  "<f>"
  dCc_de/1 -> Mux1/2  "Cc"
  ? -> Bus Selector/1
  dCD_de/1 -> Product1/2
  Bus Selector1/1 -> dCD_de/1  "<k>"
  Product1/1 -> Mux1/1  "CD"
  Bus Selector7/1 -> dCD_de/3  "<k>"
  Bus Selector7/2 -> dCD_de/4  "<f>"
  dCl_de/1 -> Mux1/4  "Cl"
  Bus Selector3/1 -> dCMy/3  "<k>"
  Bus Selector3/2 -> dCMy/4  "<f>"
  dCMy/1 -> Product3/2
  Bus Selector4/2 -> dCMy/2  "<f>"
  Bus Selector4/1 -> dCMy/1  "<k>"
  ? -> Bus Selector3/1, Bus Selector7/1
  ? -> Bus Selector4/1, Bus Selector1/1
  Bus Selector/1 -> Product3/1, Product1/1  "<Elevator>"
  Product3/1 -> Mux1/5  "Cm"
  dCn_de/1 -> Mux1/6  "Cn"
  dCL_de/1 -> Mux1/3  "CL"
  dCMy1/1 -> Mux/5
  dCn_de1/1 -> Mux/6  "Cn"
  Prelookup1/2 -> dCMy1/4, dCD_de1/4
  Alpha/1 -> Prelookup/1
  Prelookup2/1 -> dCMy1/5, dCD_de1/5
  Prelookup2/2 -> dCD_de1/6, dCMy1/6
  Prelookup1/1 -> dCMy1/3, dCD_de1/3
  Prelookup/2 -> dCMy1/2, dCD_de1/2
  dCD_de1/1 -> Mux/1
  dCL_de1/1 -> Mux/3  "CL"
  Prelookup/1 -> dCMy1/1, dCD_de1/1
  dCl_de1/1 -> Mux/4  "Cl"
  Beta/1 -> Prelookup1/1
  Actuators/1 -> Prelookup2/1
  dCc_de1/1 -> Mux/2  "Cc"
  Mux/1 -> delCoeff/1, Display/1

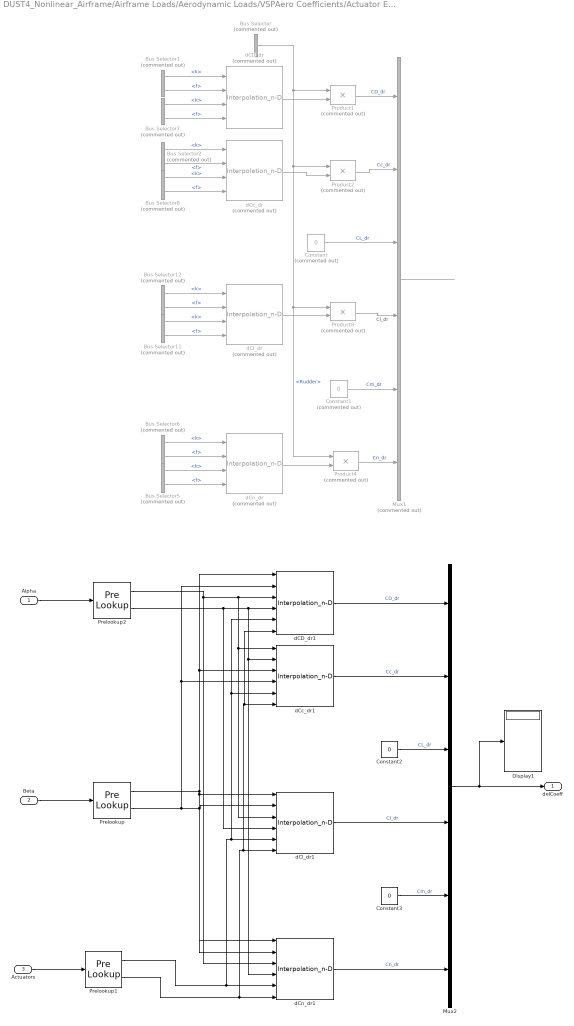
== system DUST4_Nonlinear_Airframe/Airframe Loads/Aerodynamic Loads/VSPAero Coefficients/Actuator Effects/Rudder ==
  Alpha : Inport
  Beta : Inport  Port=2
  Actuators : Inport  Port=3
  Bus Selector : BusSelector  Commented=on  OutputSignals=Rudder
  Bus Selector{1..2,5..8,11..12} (8 alike) : BusSelector  Commented=on  OutputSignals=k,f
  Constant : Constant  Commented=on  Value=0
  Constant1 : Constant  Commented=on  Value=0
  Constant2 : Constant  Value=0
  Constant3 : Constant  Value=0
  Display1 : Display
  Mux1 : Mux  Commented=on  Inputs=6
  Mux2 : Mux  Inputs=6
  Prelookup : PreLookup  BreakpointsData=Aero.beta_vec  ExtrapMethod=Linear
  Prelookup1 : PreLookup  BreakpointsData=Aero.delta_vec  ExtrapMethod=Linear
  Prelookup2 : PreLookup  BreakpointsData=Aero.alpha_vec  ExtrapMethod=Linear
  Product{1..2,4,8} (4 alike) : Product  Commented=on  InputSameDT=on  SaturateOnIntegerOverflow=on  OutDataTypeStr=Inherit: Same as first input
  dCD_dr : Interpolation_n-D  Commented=on  Table=Aero.CD_dr  RemoveProtectionIndex=on  SaturateOnIntegerOverflow=on
  dCD_dr1 : Interpolation_n-D  NumberOfTableDimensions=3  Table=Aero.CD_dr  RemoveProtectionIndex=on  SaturateOnIntegerOverflow=on
      settings: InputPortMap=u0,u1,u2,u3,u4,u5
  dCc_dr : Interpolation_n-D  Commented=on  Table=Aero.Cc_dr  RemoveProtectionIndex=on  SaturateOnIntegerOverflow=on
  dCc_dr1 : Interpolation_n-D  NumberOfTableDimensions=3  Table=Aero.Cc_dr  RemoveProtectionIndex=on  SaturateOnIntegerOverflow=on
      settings: InputPortMap=u0,u1,u2,u3,u4,u5
  dCl_dr : Interpolation_n-D  Commented=on  Table=Aero.Cl_dr  RemoveProtectionIndex=on  SaturateOnIntegerOverflow=on
  dCl_dr1 : Interpolation_n-D  NumberOfTableDimensions=3  Table=Aero.Cl_dr  RemoveProtectionIndex=on  SaturateOnIntegerOverflow=on
      settings: InputPortMap=u0,u1,u2,u3,u4,u5
  dCn_dr : Interpolation_n-D  Commented=on  Table=Aero.Cn_dr  RemoveProtectionIndex=on  SaturateOnIntegerOverflow=on
  dCn_dr1 : Interpolation_n-D  NumberOfTableDimensions=3  Table=Aero.Cn_dr  RemoveProtectionIndex=on  SaturateOnIntegerOverflow=on
      settings: InputPortMap=u0,u1,u2,u3,u4,u5
  delCoeff : Outport  VectorParamsAs1DForOutWhenUnconnected=off
  wires:
  dCc_dr/1 -> Product2/2
  Mux1/1 -> ?
  Bus Selector1/2 -> dCD_dr/2  "<f>"
  Product2/1 -> Mux1/2  "Cc_dr"
  Bus Selector2/1 -> dCc_dr/1  "<k>"
  ? -> Bus Selector/1
  dCD_dr/1 -> Product1/2
  Bus Selector2/2 -> dCc_dr/2  "<f>"
  Bus Selector1/1 -> dCD_dr/1  "<k>"
  Product1/1 -> Mux1/1  "CD_dr"
  Bus Selector7/1 -> dCD_dr/3  "<k>"
  Bus Selector7/2 -> dCD_dr/4  "<f>"
  Bus Selector8/1 -> dCc_dr/3  "<k>"
  Bus Selector8/2 -> dCc_dr/4  "<f>"
  Constant/1 -> Mux1/3  "CL_dr"
  Bus Selector11/2 -> dCl_dr/4  "<f>"
  Bus Selector11/1 -> dCl_dr/3  "<k>"
  Bus Selector12/2 -> dCl_dr/2  "<f>"
  Bus Selector12/1 -> dCl_dr/1  "<k>"
  Product8/1 -> Mux1/4  "Cl_dr"
  dCl_dr/1 -> Product8/2
  Bus Selector5/1 -> dCn_dr/3  "<k>"
  ? -> Bus Selector5/1, Bus Selector11/1, Bus Selector8/1, Bus Selector7/1
  Bus Selector5/2 -> dCn_dr/4  "<f>"
  dCn_dr/1 -> Product4/2
  ? -> Bus Selector6/1, Bus Selector12/1, Bus Selector2/1, Bus Selector1/1
  Bus Selector6/2 -> dCn_dr/2  "<f>"
  Bus Selector/1 -> Product8/1, Product4/1, Product2/1, Product1/1  "<Rudder>"
  Bus Selector6/1 -> dCn_dr/1  "<k>"
  Constant1/1 -> Mux1/5  "Cm_dr"
  Product4/1 -> Mux1/6  "Cn_dr"
  Prelookup/2 -> dCc_dr1/4, dCD_dr1/2, dCn_dr1/2, dCl_dr1/2
  Constant2/1 -> Mux2/3  "CL_dr"
  Constant3/1 -> Mux2/5  "Cm_dr"
  Prelookup2/1 -> dCn_dr1/3, dCc_dr1/1, dCl_dr1/3, dCD_dr1/3
  Prelookup1/1 -> dCD_dr1/5, dCc_dr1/5, dCl_dr1/5, dCn_dr1/5
  dCn_dr1/1 -> Mux2/6  "Cn_dr"
  dCD_dr1/1 -> Mux2/1  "CD_dr"
  dCl_dr1/1 -> Mux2/4  "Cl_dr"
  Prelookup/1 -> dCn_dr1/1, dCl_dr1/1, dCc_dr1/3, dCD_dr1/1
  Prelookup2/2 -> dCl_dr1/4, dCc_dr1/2, dCn_dr1/4, dCD_dr1/4
  dCc_dr1/1 -> Mux2/2  "Cc_dr"
  Prelookup1/2 -> dCD_dr1/6, dCc_dr1/6, dCl_dr1/6, dCn_dr1/6
  Alpha/1 -> Prelookup2/1
  Beta/1 -> Prelookup/1
  Actuators/1 -> Prelookup1/1
  Mux2/1 -> delCoeff/1, Display1/1

== system DUST4_Nonlinear_Airframe/Airframe Loads/Aerodynamic Loads/VSPAero Coefficients/Wing Rate Effects/Aero Surfaces ==
  note: C()_r
  Alpha : Inport
  Beta : Inport  Port=2
  pqr : Inport  Port=3
  V : Inport  Port=4
  Bus Creator : BusCreator  Inputs=3
  Coefs Due to Pitch Rate : Subsystem
  Coefs Due to Roll Rate : Subsystem
  Coefs Due to Yaw Rate : Subsystem
  Convert & Add : Subsystem
      settings: PortSchema="{\"entries\":[{\"content\":{\"sides\":[{\"content\":{\"connectorIds\":[\"In1\"]},\"type\":\"ConnectorPlacement.EquallySpacedRectSide\",\"uuid\":\"b8013de1-6e73-47c3-a52d-200a37bea422\"},{\"content\":{\"connectorIds\":[\"Out1\"],\"side\":\"RIGHT\"},\"type\":\"ConnectorPlacement.EquallySpacedRectSide\",\"uuid\":\"fcf5ea14-4050-433a-82d6-0b7656ed6099\"},{\"content\":{\"connectorIds\":[\"In2\",\"In3\"],\"side\":\"TOP\"},\"type\":\"ConnectorPlacement.EquallySpacedRectSide\",\"uuid\":\"1c09a769-a85c-46fb-a83d-04bd39ae92ac\"},{\"content\":{\"connectorIds\":[],\"side\":\"BOTTOM\"},\"type\":\"ConnectorPlacement.EquallySpacedRectSide\",\"uuid\":\"8f4a7c03-2c0e-435b-85d5-b3305cee738f\"}]},\"type\":\"ConnectorPlacement.EquallySpacedConnector\",\"uuid\":\"e7daaf90-0c94-4b5f-ae16-89aa994c358a\"}],\"packageUris\":[\"http://schema.mathworks.com/mf0/Connector/R2020b\"],\"version\":\"1.0\"}"
  delCoeff : Outport  VectorParamsAs1DForOutWhenUnconnected=off
  wires:
  Alpha/1 -> Coefs Due to Roll Rate/1(Alpha), Coefs Due to Yaw Rate/1(Alpha), Coefs Due to Pitch Rate/1(Alpha)
  Beta/1 -> Coefs Due to Roll Rate/2(Beta), Coefs Due to Pitch Rate/2(Beta), Coefs Due to Yaw Rate/2(Beta)
  V/1 -> Convert & Add/3(V)
  Coefs Due to Roll Rate/1(Out1) -> Bus Creator/1  "C()_p"
  Coefs Due to Pitch Rate/1(Out1) -> Bus Creator/2  "C()_q"
  pqr/1 -> Convert & Add/2(pqr)
  Bus Creator/1 -> Convert & Add/1(DampCoef)  "Damp Coef"
  Convert & Add/1(delCoeff) -> delCoeff/1
  Coefs Due to Yaw Rate/1(Out1) -> Bus Creator/3

== system DUST4_Nonlinear_Airframe/Airframe Loads/Aerodynamic Loads/VSPAero Coefficients/Wing Rate Effects/Aero Surfaces/Coefs Due to Pitch Rate ==
  note: CL_q
  note: "Flight Stability and Automatic Controls," by R. Nelson describes only 2 damping coefficients due to pitch rate. (Pg. 123): Z force, pitching moment
  Alpha : Inport
  Beta : Inport  Port=2
  Bus Selector11 : BusSelector  OutputSignals=k,f
  Bus Selector12 : BusSelector  OutputSignals=k,f
  Cm_q : Interpolation_n-D  Table=Aero.Cm_q  ExtrapMethod=Clip  RemoveProtectionIndex=on  SaturateOnIntegerOverflow=on
  Constant{,1..4} (5 alike) : Constant  Value=0
  Gain : Gain  Commented=through  Gain=0.1
  Mux1 : Mux  Inputs=6
  Out1 : Outport
  wires:
  Bus Selector11/1 -> Cm_q/3  "<k>"
  Bus Selector12/2 -> Cm_q/2  "<f>"
  Gain/1 -> Mux1/5  "Cm_q"
  Constant3/1 -> Mux1/6  "Cn_q"
  Constant1/1 -> Mux1/2  "Cc_q"
  Bus Selector12/1 -> Cm_q/1  "<k>"
  Constant2/1 -> Mux1/4  "Cl_q"
  Constant/1 -> Mux1/1  "CD_q"
  Bus Selector11/2 -> Cm_q/4  "<f>"
  Beta/1 -> Bus Selector12/1
  Alpha/1 -> Bus Selector11/1
  Mux1/1 -> Out1/1
  Cm_q/1 -> Gain/1  "CMy"
  Constant4/1 -> Mux1/3

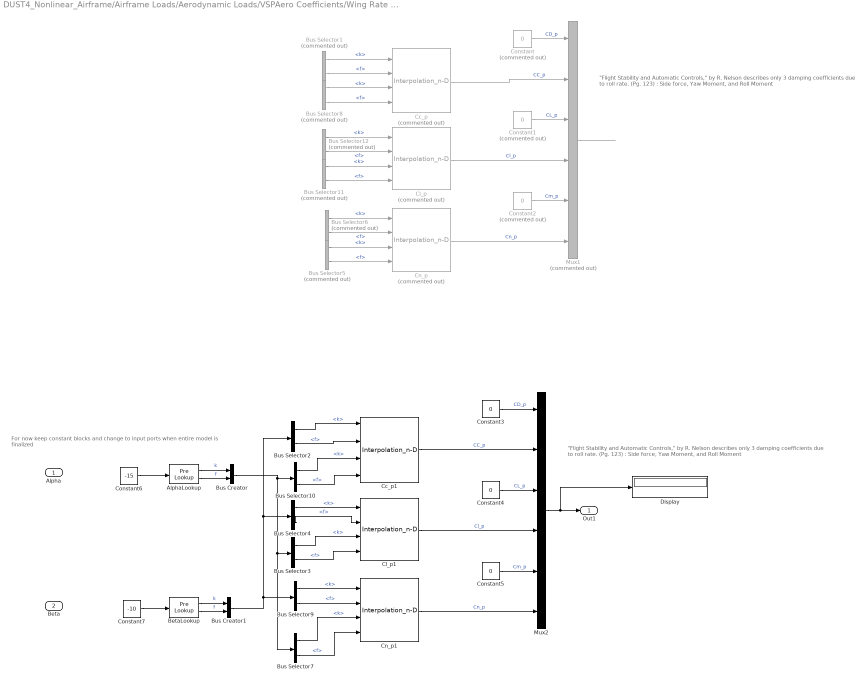
== system DUST4_Nonlinear_Airframe/Airframe Loads/Aerodynamic Loads/VSPAero Coefficients/Wing Rate Effects/Aero Surfaces/Coefs Due to Roll Rate ==
  note: "Flight Stability and Automatic Controls," by R. Nelson describes only 3 damping coefficients due to roll rate. (Pg. 123) : Side force, Yaw Moment, and Roll Moment
  note: "Flight Stability and Automatic Controls," by R. Nelson describes only 3 damping coefficients due to roll rate. (Pg. 123) : Side force, Yaw Moment, and Roll Moment
  note: For now keep
      | constant blocks and change to input ports when entire model is finalized
  Alpha : Inport
  Beta : Inport  Port=2
  AlphaLookup : PreLookup  BreakpointsData=Aero.alpha_vec  BeginIndexSearchUsingPreviousIndexResult=on  ExtrapMethod=Linear
  BetaLookup : PreLookup  BreakpointsData=Aero.beta_vec  BeginIndexSearchUsingPreviousIndexResult=on  ExtrapMethod=Linear
  Bus Creator : BusCreator  Inputs=2
  Bus Creator1 : BusCreator  Inputs=2
  Bus Selector{1,5..6,8,11..12} (6 alike) : BusSelector  Commented=on  OutputSignals=k,f
  Bus Selector{2..4,7,9..10} (6 alike) : BusSelector  OutputSignals=k,f
  Cc_p : Interpolation_n-D  Commented=on  Table=Aero.Cc_p  ExtrapMethod=Clip  RemoveProtectionIndex=on  SaturateOnIntegerOverflow=on
  Cc_p1 : Interpolation_n-D  Table=Aero.Cc_p  ExtrapMethod=Clip  RemoveProtectionIndex=on  SaturateOnIntegerOverflow=on
  Cl_p : Interpolation_n-D  Commented=on  Table=Aero.Cl_p  ExtrapMethod=Clip  RemoveProtectionIndex=on  SaturateOnIntegerOverflow=on
  Cl_p1 : Interpolation_n-D  Table=Aero.Cl_p  ExtrapMethod=Clip  RemoveProtectionIndex=on  SaturateOnIntegerOverflow=on
  Cn_p : Interpolation_n-D  Commented=on  Table=Aero.Cn_p  ExtrapMethod=Clip  RemoveProtectionIndex=on  SaturateOnIntegerOverflow=on
  Cn_p1 : Interpolation_n-D  Table=Aero.Cn_p  ExtrapMethod=Clip  RemoveProtectionIndex=on  SaturateOnIntegerOverflow=on
  Constant : Constant  Commented=on  Value=0
  Constant1 : Constant  Commented=on  Value=0
  Constant2 : Constant  Commented=on  Value=0
  Constant3 : Constant  Value=0
  Constant4 : Constant  Value=0
  Constant5 : Constant  Value=0
  Constant6 : Constant  Value=-15
  Constant7 : Constant  Value=-10
  Display : Display
  Mux1 : Mux  Commented=on  Inputs=6
  Mux2 : Mux  Inputs=6
  Out1 : Outport
  wires:
  Bus Selector11/1 -> Cl_p/3  "<k>"
  Bus Selector12/2 -> Cl_p/2  "<f>"
  Constant2/1 -> Mux1/5  "Cm_p"
  Cn_p/1 -> Mux1/6  "Cn_p"
  Cc_p/1 -> Mux1/2  "CC_p"
  Bus Selector12/1 -> Cl_p/1  "<k>"
  Bus Selector5/2 -> Cn_p/4  "<f>"
  Bus Selector8/1 -> Cc_p/3  "<k>"
  Bus Selector8/2 -> Cc_p/4  "<f>"
  Cl_p/1 -> Mux1/4  "Cl_p"
  Bus Selector6/1 -> Cn_p/1  "<k>"
  Constant/1 -> Mux1/1  "CD_p"
  Bus Selector6/2 -> Cn_p/2  "<f>"
  Bus Selector11/2 -> Cl_p/4  "<f>"
  Constant1/1 -> Mux1/3  "CL_p"
  ? -> Bus Selector6/1, Bus Selector12/1, Bus Selector1/1
  ? -> Bus Selector5/1, Bus Selector11/1, Bus Selector8/1
  Bus Selector5/1 -> Cn_p/3  "<k>"
  Mux1/1 -> ?
  Bus Selector1/1 -> Cc_p/1  "<k>"
  Bus Selector1/2 -> Cc_p/2  "<f>"
  Bus Selector10/1 -> Cc_p1/3  "<k>"
  Mux2/1 -> Display/1, Out1/1
  Bus Selector7/1 -> Cn_p1/3  "<k>"
  Constant3/1 -> Mux2/1  "CD_p"
  Constant4/1 -> Mux2/3  "CL_p"
  Bus Selector9/2 -> Cn_p1/2  "<f>"
  Cn_p1/1 -> Mux2/6  "Cn_p"
  Bus Selector3/1 -> Cl_p1/3  "<k>"
  BetaLookup/2 -> Bus Creator1/2  "f"
  AlphaLookup/1 -> Bus Creator/1  "k"
  Bus Selector7/2 -> Cn_p1/4  "<f>"
  Bus Selector9/1 -> Cn_p1/1  "<k>"
  Bus Selector10/2 -> Cc_p1/4  "<f>"
  AlphaLookup/2 -> Bus Creator/2  "f"
  Bus Selector2/2 -> Cc_p1/2  "<f>"
  Bus Selector2/1 -> Cc_p1/1  "<k>"
  Constant7/1 -> BetaLookup/1
  BetaLookup/1 -> Bus Creator1/1  "k"
  Bus Selector4/1 -> Cl_p1/1  "<k>"
  Bus Creator1/1 -> Bus Selector9/1, Bus Selector4/1, Bus Selector2/1
  Constant6/1 -> AlphaLookup/1
  Cc_p1/1 -> Mux2/2  "CC_p"
  Bus Creator/1 -> Bus Selector7/1, Bus Selector3/1, Bus Selector10/1
  Cl_p1/1 -> Mux2/4  "Cl_p"
  Bus Selector3/2 -> Cl_p1/4  "<f>"
  Bus Selector4/2 -> Cl_p1/2  "<f>"
  Constant5/1 -> Mux2/5  "Cm_p"

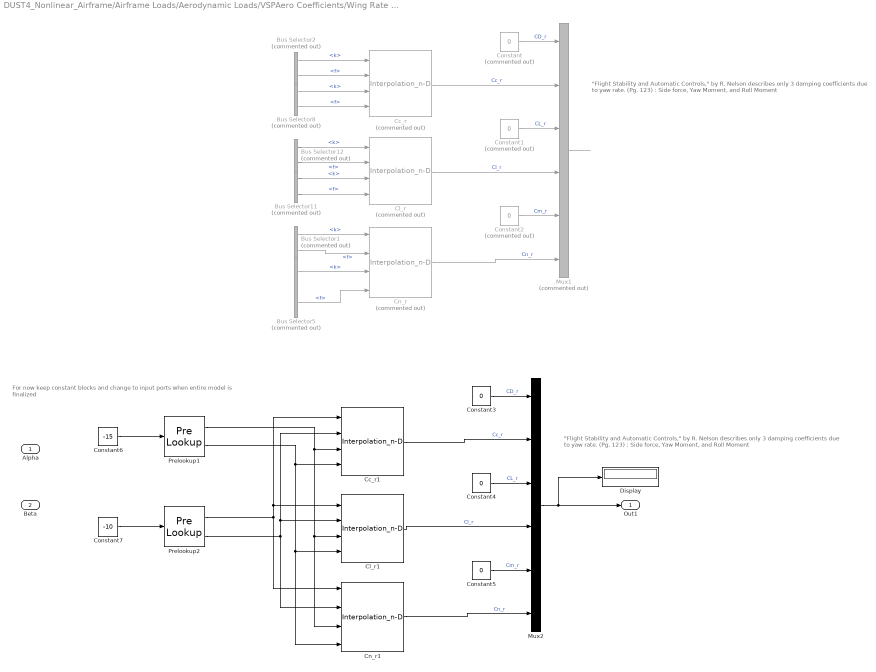
== system DUST4_Nonlinear_Airframe/Airframe Loads/Aerodynamic Loads/VSPAero Coefficients/Wing Rate Effects/Aero Surfaces/Coefs Due to Yaw Rate ==
  note: "Flight Stability and Automatic Controls," by R. Nelson describes only 3 damping coefficients due to yaw rate. (Pg. 123) : Side force, Yaw Moment, and Roll Moment
  note: "Flight Stability and Automatic Controls," by R. Nelson describes only 3 damping coefficients due to yaw rate. (Pg. 123) : Side force, Yaw Moment, and Roll Moment
  note: For now keep
      | constant blocks and change to input ports when entire model is finalized
  Alpha : Inport
  Beta : Inport  Port=2
  Bus Selector{1..2,5,8,11..12} (6 alike) : BusSelector  Commented=on  OutputSignals=k,f
  Cc_r : Interpolation_n-D  Commented=on  Table=Aero.Cc_r  ExtrapMethod=Clip  RemoveProtectionIndex=on  SaturateOnIntegerOverflow=on
  Cc_r1 : Interpolation_n-D  Table=Aero.Cc_r  ExtrapMethod=Clip  RemoveProtectionIndex=on  SaturateOnIntegerOverflow=on
  Cl_r : Interpolation_n-D  Commented=on  Table=Aero.Cl_r  ExtrapMethod=Clip  RemoveProtectionIndex=on  SaturateOnIntegerOverflow=on
  Cl_r1 : Interpolation_n-D  Table=Aero.Cl_r  ExtrapMethod=Clip  RemoveProtectionIndex=on  SaturateOnIntegerOverflow=on
  Cn_r : Interpolation_n-D  Commented=on  Table=Aero.Cn_r  ExtrapMethod=Clip  RemoveProtectionIndex=on  SaturateOnIntegerOverflow=on
  Cn_r1 : Interpolation_n-D  Table=Aero.Cn_r  ExtrapMethod=Clip  RemoveProtectionIndex=on  SaturateOnIntegerOverflow=on
  Constant : Constant  Commented=on  Value=0
  Constant1 : Constant  Commented=on  Value=0
  Constant2 : Constant  Commented=on  Value=0
  Constant3 : Constant  Value=0
  Constant4 : Constant  Value=0
  Constant5 : Constant  Value=0
  Constant6 : Constant  Value=-15
  Constant7 : Constant  Value=-10
  Display : Display
  Mux1 : Mux  Commented=on  Inputs=6
  Mux2 : Mux  Inputs=6
  Prelookup1 : PreLookup  BreakpointsData=Aero.alpha_vec  ExtrapMethod=Linear
  Prelookup2 : PreLookup  BreakpointsData=Aero.beta_vec  ExtrapMethod=Linear
  Out1 : Outport
  wires:
  Bus Selector2/1 -> Cc_r/1  "<k>"
  Bus Selector11/1 -> Cl_r/3  "<k>"
  Bus Selector12/2 -> Cl_r/2  "<f>"
  Constant2/1 -> Mux1/5  "Cm_r"
  Cn_r/1 -> Mux1/6  "Cn_r"
  Cc_r/1 -> Mux1/2  "Cc_r"
  Bus Selector12/1 -> Cl_r/1  "<k>"
  Bus Selector5/2 -> Cn_r/4  "<f>"
  Bus Selector8/1 -> Cc_r/3  "<k>"
  Bus Selector8/2 -> Cc_r/4  "<f>"
  Cl_r/1 -> Mux1/4  "Cl_r"
  Constant/1 -> Mux1/1  "CD_r"
  Bus Selector11/2 -> Cl_r/4  "<f>"
  Constant1/1 -> Mux1/3  "CL_r"
  ? -> Bus Selector1/1, Bus Selector12/1, Bus Selector2/1
  Bus Selector2/2 -> Cc_r/2  "<f>"
  ? -> Bus Selector5/1, Bus Selector11/1, Bus Selector8/1
  Bus Selector5/1 -> Cn_r/3  "<k>"
  Bus Selector1/2 -> Cn_r/2  "<f>"
  Bus Selector1/1 -> Cn_r/1  "<k>"
  Cn_r1/1 -> Mux2/6  "Cn_r"
  Mux2/1 -> Out1/1, Display/1
  Cl_r1/1 -> Mux2/4  "Cl_r"
  Constant5/1 -> Mux2/5  "Cm_r"
  Cc_r1/1 -> Mux2/2  "Cc_r"
  Constant3/1 -> Mux2/1  "CD_r"
  Constant4/1 -> Mux2/3  "CL_r"
  Constant7/1 -> Prelookup2/1
  Constant6/1 -> Prelookup1/1
  Prelookup1/1 -> Cl_r1/3, Cn_r1/3, Cc_r1/3
  Prelookup2/1 -> Cl_r1/1, Cc_r1/1, Cn_r1/1
  Prelookup2/2 -> Cn_r1/2, Cl_r1/2, Cc_r1/2
  Prelookup1/2 -> Cl_r1/4, Cn_r1/4, Cc_r1/4
  Mux1/1 -> ?
